simulink model "challenge1"  (R2025a)
settings: Solver=VariableStepAuto  StartTime=0.0  StopTime=10.0  RelTol=1e-3
undefined symbols (not defined in the file): degs2rpm, delta_c, den_Hi, K, k0, mot, num_Hi, rpm2rads, sens, w_c
settings Model: Creator=ester  LastModifiedBy=ester

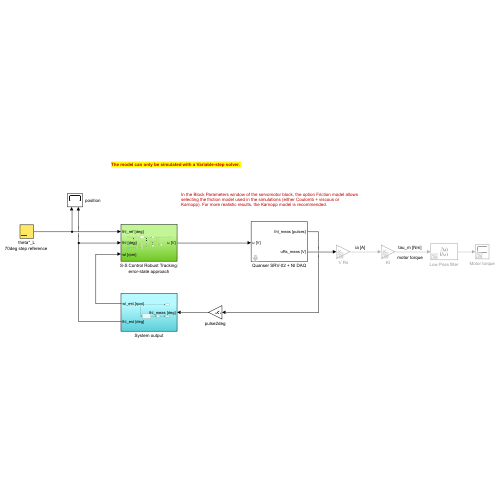
[thumbnail: Simulink's stored preview of the top-level diagram]
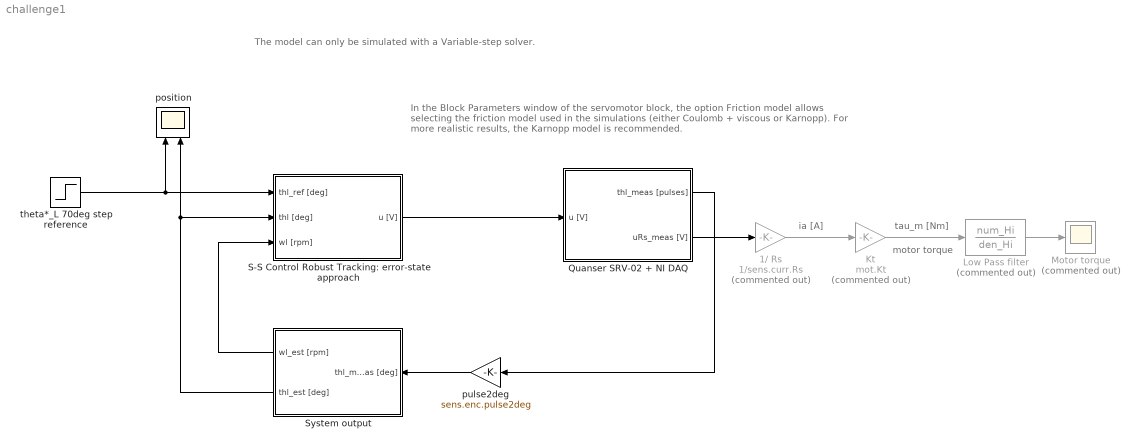
== system challenge1 ==
  note: The model can only be simulated with a Variable-step solver.
  note: In the Block Parameters window of the servomotor block, the option Friction model allows selecting the friction model used in the simulations (either Coulomb + viscous or Karnopp). For more realistic results, the Karnopp model is recommended.
  note: motor torque
  note: tau_m [Nm]
  note: ia [A]
  1/ Rs : Gain  Commented=on  Gain=1/sens.curr.Rs
  Kt : Gain  Commented=on  Gain=mot.Kt
  Low Pass filter : TransferFcn  Commented=on  Numerator=num_Hi  Denominator=den_Hi
  Motor torque : Scope  Commented=on
  Quanser SRV-02 + NI DAQ : Subsystem  mask(Quanser SRV-02 (with inertial load) + NI DAQ){Ts=0.001, fricType=Coulomb + viscous}
      mask prompts: Ts "NI DAQ Sample Time:"; fricType "Friction model"
      mask help: Quanser SRV-02 (with inertial load) + NI DAQ model.
      mask init:
      | %%  Sensors data
      | 
      | %   shunt resistor
      | sens.curr.Rs = 0.5;                         %   resistance [Ohm]   
      | sens.curr.uRs_std = 0.01;                   %   voltage noise standard dev [V]                           
      | sens.curr.uRs_var = sens.curr.uRs_std^2;	%   voltage noise variance [V^2]
      | 
      | %   Hewlett-Packard HEDS-5540#A06 optical encoder
      | sens.enc.ppr = 500*4;                       %   pulses per rotation
      | sens.enc.pulse2deg = 360/sens.enc.ppr;      %   [pulses] -> [deg]
      | sens.enc.pulse2rad = 2*pi/sens.enc.ppr;     %   [pulses] -> [rad]
      | sens.enc.deg2pulse = sens.enc.ppr/360;      %   [deg] -> [pulses]
      | sens.enc.rad2pulse = sens.enc.ppr/2/pi;     %   [rad] -> [pulses]
      | 
      | 
      | %%  Data acquisition board (daq) data
      | 
      | %   NI PCI-6221 DAC data
      | daq.dac.bits = 16;                                  %   resolution (bits)
      | daq.dac.fs   = 10;                                  %   full scale 
      | daq.dac.q    = 2*daq.dac.fs/(2^daq.dac.bits-1);     %	quantization
      | 
      | %   NI PCI-6221 ADC data
      | daq.adc.bits = 16;                                  %   resolution (bits)
      | daq.adc.fs   = 10;                                  %   full scale (as set in SLDRT Analog Input block)
      | daq.adc.q    = 2*daq.adc.fs/(2^daq.adc.bits-1);     %   quantization
      mask Help:
      | Riccardo Antonello (antonello@dei.unipd.it)
      | 
      | April 24, 2020
      | 
      | Dept. of Information Engineering, University of Padova
      mask TypeOptions fricType: Coulomb + viscous | Karnopp
  S-S Control Robust Tracking: error-state approach : Subsystem
  System output : Subsystem
  position : Scope  NumInputPorts=2
      settings: ActiveDisplayYMinimum=68.584768073085527  ActiveDisplayYMaximum=70.433956532127965
  pulse2deg : Gain  Gain=sens.enc.pulse2deg
  "theta*_L 70deg step reference " : Step  Time=0  After=70  SampleTime=0
  wires:
  System output/1(wl_est [rpm]) -> S-S Control Robust Tracking: error-state approach/3(wl [rpm])
  "theta*_L 70deg step reference "/1 -> S-S Control Robust Tracking: error-state approach/1(thl_ref [deg]), position/1
  System output/2(thl_est [deg]) -> S-S Control Robust Tracking: error-state approach/2(thl [deg]), position/2
  pulse2deg/1 -> System output/1(thl_meas [deg])
  S-S Control Robust Tracking: error-state approach/1(u [V]) -> Quanser SRV-02 + NI DAQ/1(u [V])
  Quanser SRV-02 + NI DAQ/1(thl_meas [pulses]) -> pulse2deg/1
  1/ Rs/1 -> Kt/1
  Low Pass filter/1 -> Motor torque/1
  Kt/1 -> Low Pass filter/1
  Quanser SRV-02 + NI DAQ/2(uRs_meas [V]) -> 1/ Rs/1

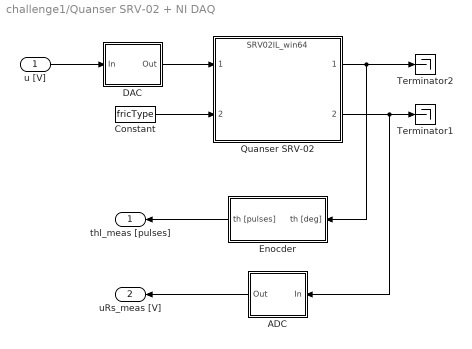
== system challenge1/Quanser SRV-02 + NI DAQ ==
  u [V] : Inport
  ADC : Subsystem
  Constant : Constant  Value=fricType
  DAC : Subsystem
  Enocder : Subsystem
  Quanser SRV-02 : ModelReference  ModelNameDialog=SRV02IL_win64.slxp  ModelReferenceVersion=1.44  CopyOfModelProtected=on
  Terminator1 : Terminator
  Terminator2 : Terminator
  thl_meas [pulses] : Outport
  uRs_meas [V] : Outport  Port=2
  wires:
  Enocder/1(th [pulses]) -> thl_meas [pulses]/1
  ADC/1(Out) -> uRs_meas [V]/1
  DAC/1(Out) -> Quanser SRV-02/1
  Quanser SRV-02/2 -> ADC/1(In), Terminator1/1
  u [V]/1 -> DAC/1(In)
  Quanser SRV-02/1 -> Enocder/1(th [deg]), Terminator2/1
  Constant/1 -> Quanser SRV-02/2

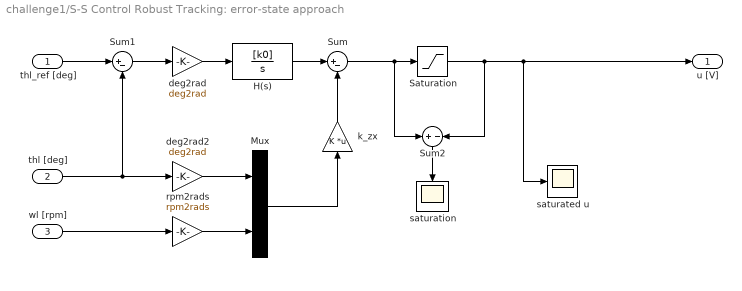
== system challenge1/S-S Control Robust Tracking: error-state approach ==
  thl_ref [deg] : Inport
  thl [deg] : Inport  Port=2
  wl [rpm] : Inport  Port=3
  H(s) : TransferFcn  Numerator=[k0]  Denominator=[1 0]
  Mux : Mux  Inputs=2
  Saturation : Saturate  UpperLimit=10  LowerLimit=-10  ZeroCross=off
  Sum : Sum  Inputs=|+-
  Sum1 : Sum  Inputs=|+-
  Sum2 : Sum  Inputs=+-
  deg2rad : Gain  Gain=deg2rad
  deg2rad2 : Gain  Gain=deg2rad
  k_zx : Gain  Gain=K  Multiplication=Matrix(K*u)
  rpm2rads : Gain  Gain=rpm2rads
  saturated u : Scope
      settings: ActiveDisplayYMinimum=-1.1813619039912078  ActiveDisplayYMaximum=5.14904278969362  DataLoggingVariableName=ScopeData2
  saturation : Scope
      settings: ActiveDisplayYMinimum=-0.17005917159763317  ActiveDisplayYMaximum=0.0906745562130177  DataLoggingVariableName=ScopeData3
  u [V] : Outport
  wires:
  deg2rad2/1 -> Mux/1
  rpm2rads/1 -> Mux/2
  Saturation/1 -> Sum2/2, u [V]/1, saturated u/1
  thl [deg]/1 -> Sum1/2, deg2rad2/1
  wl [rpm]/1 -> rpm2rads/1
  Mux/1 -> k_zx/1
  k_zx/1 -> Sum/2
  Sum/1 -> Sum2/1, Saturation/1
  deg2rad/1 -> H(s)/1
  H(s)/1 -> Sum/1
  thl_ref [deg]/1 -> Sum1/1
  Sum1/1 -> deg2rad/1
  Sum2/1 -> saturation/1

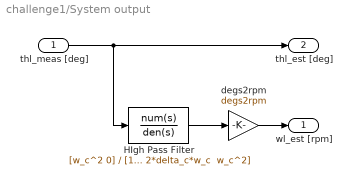
== system challenge1/System output ==
  thl_meas [deg] : Inport
  HIgh Pass Filter : TransferFcn  Numerator=[w_c^2 0]  Denominator="[1 2*delta_c*w_c  w_c^2]"
  degs2rpm : Gain  Gain=degs2rpm
  wl_est [rpm] : Outport
  thl_est [deg] : Outport  Port=2
  wires:
  thl_meas [deg]/1 -> HIgh Pass Filter/1, thl_est [deg]/1
  HIgh Pass Filter/1 -> degs2rpm/1
  degs2rpm/1 -> wl_est [rpm]/1

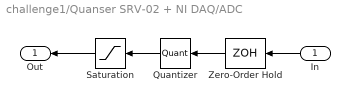
== system challenge1/Quanser SRV-02 + NI DAQ/ADC ==
  In : Inport
  Quantizer : Quantizer  QuantizationInterval=daq.adc.q
  Saturation : Saturate  UpperLimit=daq.adc.fs  LowerLimit=-daq.adc.fs
  Zero-Order Hold : ZeroOrderHold  SampleTime=Ts
  Out : Outport
  wires:
  Saturation/1 -> Out/1
  In/1 -> Zero-Order Hold/1
  Quantizer/1 -> Saturation/1
  Zero-Order Hold/1 -> Quantizer/1

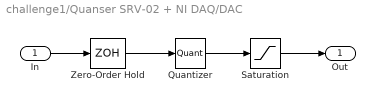
== system challenge1/Quanser SRV-02 + NI DAQ/DAC ==
  In : Inport
  Quantizer : Quantizer  QuantizationInterval=daq.dac.q
  Saturation : Saturate  UpperLimit=daq.dac.fs  LowerLimit=-daq.dac.fs
  Zero-Order Hold : ZeroOrderHold  SampleTime=Ts
  Out : Outport
  wires:
  Quantizer/1 -> Saturation/1
  In/1 -> Zero-Order Hold/1
  Zero-Order Hold/1 -> Quantizer/1
  Saturation/1 -> Out/1

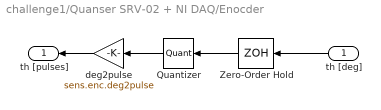
== system challenge1/Quanser SRV-02 + NI DAQ/Enocder ==
  th [deg] : Inport
  Quantizer : Quantizer  QuantizationInterval=sens.enc.pulse2deg
  Zero-Order Hold : ZeroOrderHold  SampleTime=Ts
  deg2pulse : Gain  Gain=sens.enc.deg2pulse
  th [pulses] : Outport
  wires:
  Quantizer/1 -> deg2pulse/1
  th [deg]/1 -> Zero-Order Hold/1
  Zero-Order Hold/1 -> Quantizer/1
  deg2pulse/1 -> th [pulses]/1
